simulink model "fcev_model_ssc"  (R2023a)
settings: Solver=VariableStepAuto  StartTime=0.0  StopTime=2474  RelTol=1e-3
model workspace (MAT data in the model file):
  N_P0 = 3
libraries: nesl_utility x12, fl_lib x7, sdl_lib x6, ee_lib x2, autolibshared x2, slpidlib x2, autolibdatasheetbattery x1, simulink x1, autolibmappedmotor x1
settings Model: Creator=connl  LastModifiedBy=connl
settings SolverCC: MaxConsecutiveMinStep=5  DaesscMode=Robust  SolverResetMethod=Robust
settings DebuggingCC: AlgebraicLoopMsg=none

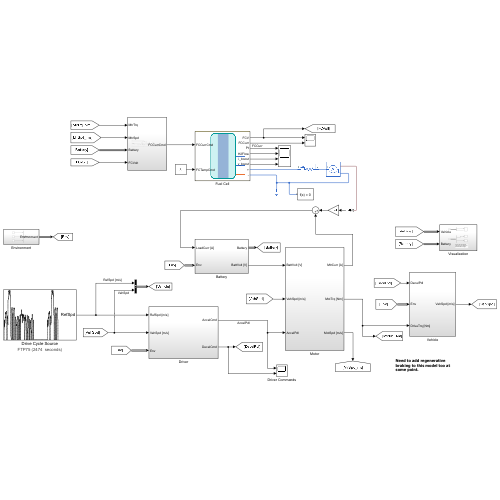
[thumbnail: Simulink's stored preview of the top-level diagram]
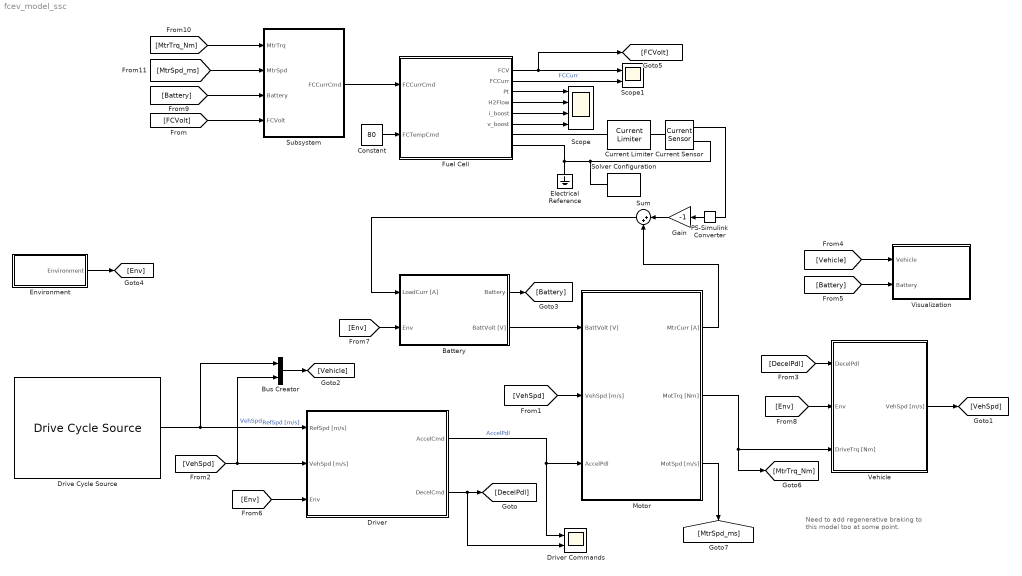
== system fcev_model_ssc ==
  note: Need to add regenerative braking to this model too at some point.
  Battery : Subsystem
  Bus Creator : BusCreator  Inputs=2
  Constant : Constant  Value=80
  Current Limiter : ee_lib/Semiconductors & Converters/Current Limiter  iLim=25 A  vLim=0.1 V  gLim=1e-3 1/Ohm  thermal_mass=100 J/K  initial_temperature=298.15 K
      settings: InternalSimscapePortConfiguration="{\"Bottom\":[],\"Left\":[{\"id\":\"p\",\"label\":\"+\",\"type\":\"foundation.electrical.electrical\"}],\"Right\":[{\"id\":\"n\",\"label\":\"-\",\"type\":\"foundation.electrical.electrical\"}],\"Top\":[]}"
  Current Sensor : fl_lib/Electrical/Electrical Sensors/Current Sensor
  Drive Cycle Source : autolibshared/Drive Cycle Source  cycleVar=FTP75  fileVar=cycleFTP75.mat  tfinal="2474  seconds"  cycleRepeat=off  outAccPort=off  outGearPort=off  gearList=No gear data  t_wot1=5  xdot_woto=0  xdot_wot1=30  t_wot2=20  xdot_wot2=0  t_wotend=30  srcUnit=m/s  outUnit=m/s  srcAccUnit=m/s/s  outAccUnit=m/s^2  dt=0  aMode=1  faultOption=off  velBnd=2  velBndUnit=mph  inUnit=m/s  timeBnd=1  failOption=off  stopSim=off  maxFaultCnt=10  maxFaultTime=2  maxTotFaultTime=15  traceOption=off  dtTrace=1  traceWindow=10  lastDCname=FTP75  lastOutUnit=mph  lastDT=0  lastTB=1  lastSB=2  forceCalcBound=off
  Driver : Subsystem
  Driver Commands : Scope  NumInputPorts=2
  Electrical Reference : fl_lib/Electrical/Electrical Elements/Electrical Reference
  Environment : Subsystem
  Fuel Cell : Subsystem  VariantControl=0
      mask Display: image('fuel_cell_converter_IMAGE.png'); % Use "Edit Image" on toolstrip to change.
  Gain : Gain  Gain=-1
  Motor : Subsystem
  PS-Simulink Converter : nesl_utility/PS-Simulink Converter  PhysicalDomain=network_engine_domain  SubClassName=ps_output  LeftPortType=input  RightPortType=output  PseudoPeriodic=off  Frequencies=[]  VectorFormat=inherit  Unit=inherit  AffineConversion=off
  Scope : Scope  NumInputPorts=4
  Scope1 : Scope  NumInputPorts=2
  Solver Configuration : nesl_utility/Solver Configuration  PhysicalDomain=network_engine_domain  SubClassName=solver  LeftPortType=input  RightPortType=generic  Tones=[]  Harmonics=[]  SimulateNoise=off  Profile=off  UseLocalSampling=off  EnableSwitchedLinearOptims=on  FrequencyDomain=off  UseCCode=off  RelTol=0.001  AbsTol=0.001  MinStep=1e-09  ToWorkspace=off  RevertToSquareIcSolve=off  NumHomotopyIterations=100  PhasorMode=off  PhasorModeNumHarmonics=1  ConsistencySolver=NEWTON_XTOL_AFTER_FTOL  IndexReductionMethod=DerivativeReplacement  DoDC=off  ResidualTolerance=1e-09  ConsistencyTolSource=GLOBAL  ConsistencyAbsTol=0.001  ConsistencyRelTol=0.001  ConsistencyTolFactor=0.001  UseLocalSolver=off  LocalSolverChoice=NE_BACKWARD_EULER_ADVANCER  ResolveIndetEquations=on  FunctionEvalNumThread=1  LocalSolverSampleTime=0.001  DoFixedCost=off  MaxNonlinIter=3  MaxModeIter=2  ComputeImpulses=off  ImpulseIterations=2  LinearAlgebra=auto  LinearAlgebraNumThread=0  EquationFormulation=NE_TIME_EF  DelaysMemoryBudget=1024  AutomaticFiltering=on  FilteringTimeConstant=0.001  PartitionStorageMethod=AS_NEEDED  PartitionMemoryBudget=1024  PartitionMethod=ROBUST
  Subsystem : Subsystem
  Sum : Sum  Inputs=|++
  Vehicle : Subsystem
  Visualization : Subsystem
  wires:
  Drive Cycle Source/1 -> Driver/1(RefSpd [m/s]), Bus Creator/1  "RefSpd [m/s]"
  Battery/2(BattVolt [V]) -> Motor/1(BattVolt [V])
  [VehSpd] -> Motor/2(VehSpd [m/s])
  [VehSpd] -> Driver/2(VehSpd [m/s]), Bus Creator/2  "VehSpd"
  [DecelPdl] -> Vehicle/1(DecelPdl)
  Vehicle/1(VehSpd [m/s]) -> [VehSpd]
  Bus Creator/1 -> [Vehicle]
  [Vehicle] -> Visualization/1(Vehicle)
  [Battery] -> Visualization/2(Battery)
  Environment/1(Environment) -> [Env]
  Battery/1(Battery) -> [Battery]
  Driver/1(AccelCmd) -> Driver Commands/1, Motor/3(AccelPdl)  "AccelPdl"
  Driver/2(DecelCmd) -> Driver Commands/2, [DecelPdl]
  [Env] -> Battery/2(Env)
  [Env] -> Driver/3(Env)
  [Env] -> Vehicle/2(Env)
  Motor/1(MtrCurr [A]) -> Sum/2
  Motor/2(MotTrq [Nm]) -> [MtrTrq_Nm], Vehicle/3(DriveTrq [Nm])
  Fuel Cell/4(H2Flow) -> Scope/2
  Fuel Cell/5(i_boost) -> Scope/3
  Fuel Cell/6(v_boost) -> Scope/4
  Fuel Cell/2(FCCurr) -> Scope1/2  "FCCurr"
  Sum/1 -> Battery/1(LoadCurr [A])
  Fuel Cell/3(Pt) -> Scope/1
  Fuel Cell/1(FCV) -> [FCVolt], Scope1/1
  Constant/1 -> Fuel Cell/2(FCTempCmd)
  Motor/3(MotSpd [m/s]) -> [MtrSpd_ms]
  [MtrTrq_Nm] -> Subsystem/1(MtrTrq)
  [MtrSpd_ms] -> Subsystem/2(MtrSpd)
  [Battery] -> Subsystem/3(Battery)
  [FCVolt] -> Subsystem/4(FCVolt)
  Subsystem/1(FCCurrCmd) -> Fuel Cell/1(FCCurrCmd)
  PS-Simulink Converter/1 -> Gain/1
  Gain/1 -> Sum/1
  connections:
  Fuel Cell/RConn1 -- Current Limiter/LConn1
  Fuel Cell/RConn2 -- Current Sensor/RConn2 -- Solver Configuration/RConn1 -- Electrical Reference/LConn1
  Current Sensor/RConn1 -- PS-Simulink Converter/LConn1
  Current Limiter/RConn1 -- Current Sensor/LConn1

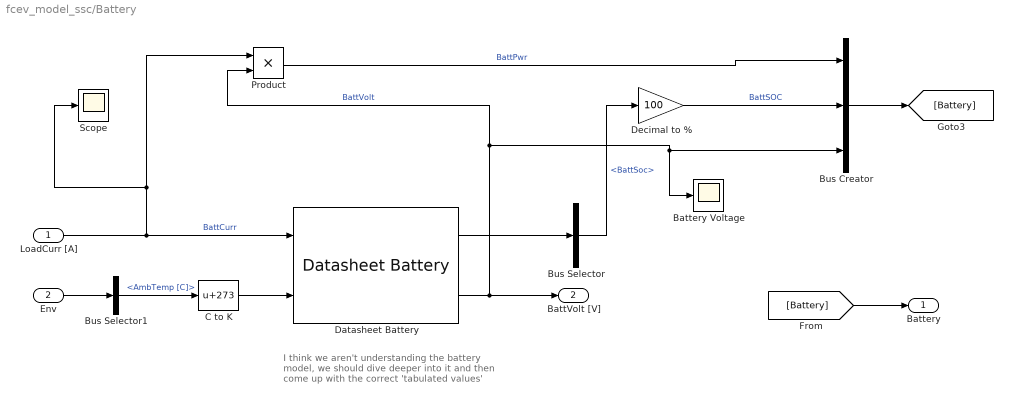
== system fcev_model_ssc/Battery ==
  note: I think we aren't understanding the battery model, we should dive deeper into it and then come up with the correct 'tabulated values'
  LoadCurr [A] : Inport
  Env : Inport  Port=2
  Battery Voltage : Scope
  Bus Creator : BusCreator  Inputs=3
  Bus Selector : BusSelector  OutputSignals=BattSoc
  Bus Selector1 : BusSelector  OutputSignals=AmbTemp [C]
  C to K : Bias  Bias=273  SaturateOnIntegerOverflow=off
  Datasheet Battery : autolibdatasheetbattery/Datasheet Battery  CapacityCtrl=Parameter  OutputVlt=Unfiltered  BattChargeMax=16  Em=[2.8 3.228 3.284 3.361 3.408 3.427 3.472 3.477 3.493 3.504 3.516 3.528 3.537 3.545 3.555 3.561 3.566 3.576 3.587 3.589 3.594 3.6 3.608 3.61 3.616 3.619 3.626 3.632 3.637 3.64 3.645 3.646 3.652 3.655 3.658 3.661 3.664 3.668 3.673 3.678 3.68 3.681 3.686 3.692 3.699 3.702 3.705 3.71 3.717 3.723 3.728 3.733 3.735 3.742 3.749 3.755 3.761 3.768 3.773 3.78 3.791 3.798 3.798 3.814 3.818 3.825 3.841 3.846 3.855 3.863 3.877 3.885 3.894 3.907 3.919 3.926 3.935 3.944 3.954 3.964 3.974 3.988 3.998 4.014 4.029 4.034 4.047 4.065 4.074 4.086 4.097 4.131 4.126 4.138 4.15 4.18 4.174 4.187 4.207 4.231 4.221]  CapLUTBp=[0 0.01 0.02 0.03 0.04 0.05 0.06 0.07 0.08 0.09 0.1 0.11 0.12 0.13 0.14 0.15 0.16 0.17 0.18 0.19 0.2 0.21 0.22 0.23 0.24 0.25 0.26 0.27 0.28 0.29 0.3 0.31 0.32 0.33 0.34 0.35 0.36 0.37 0.38 0.39 0.4 0.41 0.42 0.43 0.44 0.45 0.46 0.47 0.48 0.49 0.5 0.51 0.52 0.53 0.54 0.55 0.56 0.57 0.58 0.59 0.6 0.61 0.62 0.63 0.64 0.65 0.66 0.67 0.68 0.69 0.7 0.71 0.72 0.73 0.74 0.75 0.76 0.77 0.78 0.79 0.8 0.81 0.82 0.83 0.84 0.85 0.86 0.87 0.88 0.89 0.9 0.91 0.92 0.93 0.94 0.95 0.96 0.97 0.98 0.99 1]  RInt=0.001*[1, 1, 1, 1, 1, 1;1, 1, 1, 1, 1, 1]  BattTempBp=[240, 320]  CapSOCBp=[0 0.2 0.4 0.6 0.8 1]  Ns=12  Np=2  BattCapInit=32  Tc=1/1000  Vinit=4.221  RefBlkName='autolibdatasheetbattery/Datasheet Battery'
  Decimal to % : Gain  Gain=100
  Product : Product
  Scope : Scope
  Battery : Outport
  BattVolt [V] : Outport  Port=2
  wires:
  C to K/1 -> Datasheet Battery/2
  Datasheet Battery/1 -> Bus Selector/1
  Bus Selector/1 -> Decimal to %/1  "<BattSoc>"
  Decimal to %/1 -> Bus Creator/2  "BattSOC"
  Datasheet Battery/2 -> BattVolt [V]/1, Product/2, Bus Creator/3, Battery Voltage/1  "BattVolt"
  [Battery] -> Battery/1
  Env/1 -> Bus Selector1/1
  Bus Selector1/1 -> C to K/1  "<AmbTemp [C]>"
  Product/1 -> Bus Creator/1  "BattPwr"
  LoadCurr [A]/1 -> Scope/1, Product/1, Datasheet Battery/1  "BattCurr"
  Bus Creator/1 -> [Battery]

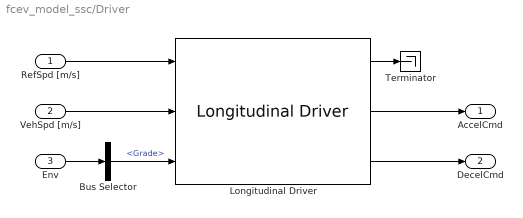
== system fcev_model_ssc/Driver ==
  RefSpd [m/s] : Inport
  VehSpd [m/s] : Inport  Port=2
  Env : Inport  Port=3
  Bus Selector : BusSelector  OutputSignals=Grade
  Longitudinal Driver : autolibshared/Longitudinal Driver  extAccelOvr=off  extDecelOvr=off  extAccelHld=off  extDecelHld=off  extAccelZero=off  extDecelZero=off  cntrlType=PI  shftType=None  velUnits=m/s  gearOut=off  Kp=20  Ki=1  Kff=.05  Kg=.01  VehVelVec=[0 100]  KffVec=[.1 .1]  KpVec=[10 10]  KiVec=[5 5]  KgVec=[0 0]  m=1500  Kpt=3000  tau=.1  L=2  aR=200  bR=2.5  cR=.5  g=9.81  vnom=100  Kaw=.1  tauerr=.03  tauPt=2  GearInit=0  tShift=.1  pdlVec=[0.1 0.4 0.5 0.9]  upShftTbl=[-1 12.9375 26.4375 39.9375 51.18749999999999 62.4375 72.84375 83.25;-1 16.3125 29.8125 43.3125 54.5624 65.8125 76.78125 87.75;-1 19.6875 33.1875 46.68749999999999 57.9375 69.1875 80.71875 92.25;-1 33 52.5 77.25 100.5 138.75 161.875 185]  dwnShftTbl=[1 9.5625 23.0625 36.5625 47.8125 59.0625 68.90625 78.75;1 12.9375 26.4375 39.9375 51.18749999999999 62.4375 72.84375 83.25;1 16.3125 29.8125 43.3125 54.562499 65.8125 76.78125 87.75;1 19.6875 33.1875 46.68749999999999 57.9375 69.1875 80.71875 92.25]  tClutch=.5  tRev=.5  tPark=120  aMode=1  UpGearVec="[0  1  2  3  4  5  6  7]"  DownGearVec="[1  2  3  4  5  6  7  8]"
  Terminator : Terminator
  AccelCmd : Outport
  DecelCmd : Outport  Port=2
  wires:
  VehSpd [m/s]/1 -> Longitudinal Driver/2
  Longitudinal Driver/2 -> AccelCmd/1
  RefSpd [m/s]/1 -> Longitudinal Driver/1
  Bus Selector/1 -> Longitudinal Driver/3  "<Grade>"
  Env/1 -> Bus Selector/1
  Longitudinal Driver/3 -> DecelCmd/1
  Longitudinal Driver/1 -> Terminator/1

== system fcev_model_ssc/Environment ==
  AmbTemp : Constant  Value=25
  Bus Creator : BusCreator  Inputs=3
  Grade : Constant  Value=0
  WindSpdx : Constant  Value=0
  Environment : Outport
  wires:
  Grade/1 -> Bus Creator/1  "Grade"
  WindSpdx/1 -> Bus Creator/2  "WindSpdx [m/s]"
  AmbTemp/1 -> Bus Creator/3  "AmbTemp [C]"
  Bus Creator/1 -> Environment/1

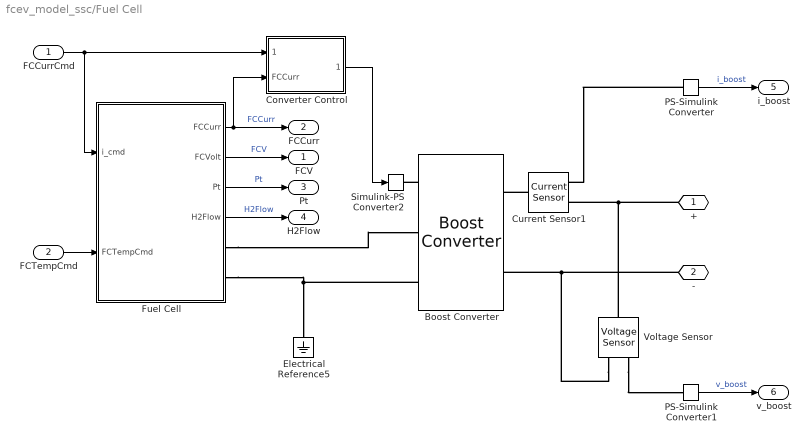
== system fcev_model_ssc/Fuel Cell ==
  FCCurrCmd : Inport
  FCTempCmd : Inport  Port=2
  Boost Converter : ee_lib/Semiconductors & Converters/Converters/Boost Converter  port_option=ee.enum.controlport.ps  device_type=ee.enum.converters.switchingdevice.averaged  Vf=0.8 V  Ron=0.001 Ohm  Rds=0.001 Ohm  Goff=1e-5 1/Ohm  Vgt=1 V  Vgt_off=-1 V  Ih=1 A  Vth=6 V  K=0  diode_param=ee.enum.converters.diode.nodynamics  diode_Vf=0.8 V  diode_Ron=0.001 Ohm  diode_Goff=1e-05 1/Ohm  diode_C=50 nF  diode_iRM=-235 A  diode_iF=300 A  diode_idot=-50 A/us  diode_trr_param=ee.enum.converters.diodetrr.trr_factor  diode_trr_factor=3  diode_trr=15 us  diode_Qrr=1500 s*uA  Lf=0.005 H  Rl=0 Ohm  Cf=0.001 F  Rf=10 Ohm  snubber_type=ee.enum.converters.snubber.exclude  Cs=1e-7 F  Rs=0.1 Ohm  iL_specify=on  iL_priority=High  iL=0 A  iL_nominal_specify=off  iL_nominal_unit=A  iL_nominal_value=1  vc_specify=on  vc_priority=High  vc=650 V  vc_nominal_specify=off  vc_nominal_unit=V  vc_nominal_value=1
      settings: InternalSimscapePortConfiguration="{\"Bottom\":[],\"Left\":[{\"id\":\"G\",\"label\":\"G\",\"type\":\"input\"},{\"id\":\"p1\",\"label\":\"1+\",\"type\":\"foundation.electrical.electrical\"},{\"id\":\"n1\",\"label\":\"1-\",\"type\":\"foundation.electrical.electrical\"}],\"Right\":[{\"id\":\"p2\",\"label\":\"2+\",\"type\":\"foundation.electrical.electrical\"},{\"id\":\"n2\",\"label\":\"2-\",\"type\":\"foundation.electrical.electrical\"}],\"Top\":[]}"
  Converter Control : Subsystem
  Current Sensor1 : fl_lib/Electrical/Electrical Sensors/Current Sensor
  Electrical Reference5 : fl_lib/Electrical/Electrical Elements/Electrical Reference
  Fuel Cell : Subsystem  Variant=on  VariantControlMode=label  VariantControl=Choice  LabelModeActiveChoice=SimscapeFuelCell
  PS-Simulink Converter : nesl_utility/PS-Simulink Converter  PhysicalDomain=network_engine_domain  SubClassName=ps_output  LeftPortType=input  RightPortType=output  PseudoPeriodic=off  Frequencies=[]  VectorFormat=inherit  Unit=inherit  AffineConversion=off
  PS-Simulink Converter1 : nesl_utility/PS-Simulink Converter  PhysicalDomain=network_engine_domain  SubClassName=ps_output  LeftPortType=input  RightPortType=output  PseudoPeriodic=off  Frequencies=[]  VectorFormat=inherit  Unit=inherit  AffineConversion=off
  Simulink-PS Converter2 : nesl_utility/Simulink-PS Converter  PhysicalDomain=network_engine_domain  SubClassName=ps_input  LeftPortType=input  RightPortType=output  PseudoPeriodic=off  Frequencies=[]  NoiseDistribution=none  NoiseParameters=[]  Unit=1  AffineConversion=off  FilteringAndDerivatives=provide  SimscapeFilterOrder=1  InputFilterTimeConstant=0.001  UdotUserProvided=0
  Voltage Sensor : fl_lib/Electrical/Electrical Sensors/Voltage Sensor
  + : PMIOPort  Side=Right
  - : PMIOPort  Port=2  Side=Right
  FCV : Outport
  FCCurr : Outport  Port=2
  Pt : Outport  Port=3
  H2Flow : Outport  Port=4
  i_boost : Outport  Port=5
  v_boost : Outport  Port=6
  wires:
  Converter Control/1(u_boost) -> Simulink-PS Converter2/1
  Fuel Cell/1(FCCurr) -> FCCurr/1, Converter Control/2(FCCurr)  "FCCurr"
  FCCurrCmd/1 -> Fuel Cell/1(i_cmd), Converter Control/1(FCCurrCmd)
  FCTempCmd/1 -> Fuel Cell/2(FCTempCmd)
  Fuel Cell/2(FCVolt) -> FCV/1  "FCV"
  Fuel Cell/3(Pt) -> Pt/1  "Pt"
  Fuel Cell/4(H2Flow) -> H2Flow/1  "H2Flow"
  PS-Simulink Converter/1 -> i_boost/1  "i_boost"
  PS-Simulink Converter1/1 -> v_boost/1  "v_boost"
  connections:
  Boost Converter/LConn1 -- Simulink-PS Converter2/RConn1
  -/RConn1 -- Voltage Sensor/RConn2 -- Boost Converter/RConn2
  +/RConn1 -- Voltage Sensor/LConn1 -- Current Sensor1/RConn2
  Current Sensor1/LConn1 -- Boost Converter/RConn1
  Boost Converter/LConn3 -- Fuel Cell/RConn2 -- Electrical Reference5/LConn1
  PS-Simulink Converter/LConn1 -- Current Sensor1/RConn1
  Fuel Cell/RConn1 -- Boost Converter/LConn2
  Voltage Sensor/RConn1 -- PS-Simulink Converter1/LConn1

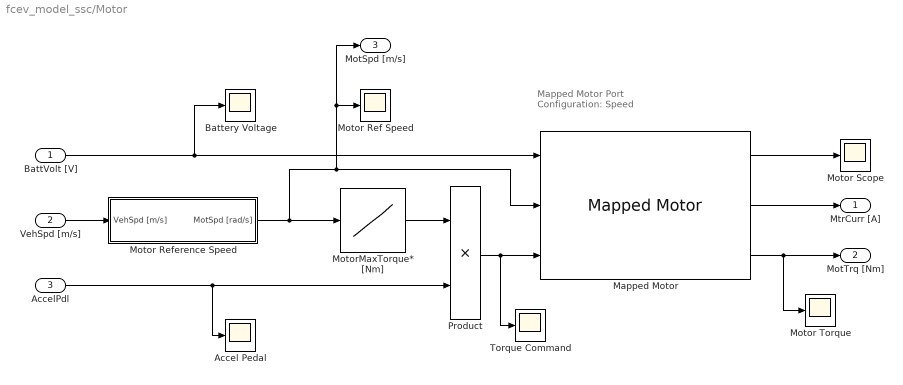
== system fcev_model_ssc/Motor ==
  note: Mapped Motor
      | Port Configuration: Speed
  BattVolt [V] : Inport
  VehSpd [m/s] : Inport  Port=2
  AccelPdl : Inport  Port=3
  Accel Pedal : Scope
  Battery Voltage : Scope
  Mapped Motor : autolibmappedmotor/Mapped Motor  port_config=Speed  param_by=Tabulated torque-speed envelope  w_t=[0, 100, 200, 300, 400, 500, 600]  T_t=[85, 85, 85, 80, 70, 55, 30]  torque_max=110  power_max=21000  Tc=0.02  param_loss=Single efficiency measurement  eff=90  w_eff=400  T_eff=55  Piron=0  Pbase=0  w_eff_bp=[-800 -400 0 400 800]  T_eff_bp=[0 0.03 0.06 0.09]  Temp_eff_bp=[233.15 293.15 373.15]  losses_table=[1.49 1.67 2.21 3.10; 0.42 0.69 1.14 2.03; 0.06 0.24 0.78 1.68; 0.42 0.69 1.14 2.03; 1.49 1.67 2.21 3.10]  losses_table_3d=cat(3,[1.49 1.67 2.21 3.10; 0.42 0.69 1.14 2.03; 0.06 0.24 0.78 1.68; 0.42 0.69 1.14 2.03; 1.49 1.67 2.21 3.10],[1.49 1.67 2.21 3.10; 0.42 0.69 1.14 2.03; 0.06 0.24 0.78 1.68; 0.42 0.69 1.14 2.03; 1.49 1.67 2.21 3.10],[1.49 1.67 2.21 3.10; 0.42 0.69 1.14 2.03; 0.06 0.24 0.78 1.68; 0.42 0.69 1.14 2.03; 1.49 1.67 2.21 3.10])  efficiency_table=[95 95 95 95; 95 95 95 95; 95 95 95 95; 95 95 95 95; 95 95 95 95]  efficiency_table_3d=cat(3,[95 95 95 95; 95 95 95 95; 95 95 95 95; 95 95 95 95; 95 95 95 95],[95 95 95 95; 95 95 95 95; 95 95 95 95; 95 95 95 95; 95 95 95 95],[95 95 95 95; 95 95 95 95; 95 95 95 95; 95 95 95 95; 95 95 95 95])  J=5e-6  b=1e-5  omega_o=0  T_t_extended=[30 55 70 80 85 85 85 85 85 80 70 55 30]  w_t_extended=[-600 -500 -400 -300 -200 -100 0 100 200 300 400 500 600]  KLossIron=0  KLossCopper=0.80808  x_w_eff_vec=[-8000 -4000 0 4000 8000]  x_T_eff_vec=[-0.09 -0.06 -0.03 0 0.03 0.06 0.09]  x_tmp_eff_vec=[-0.09 -0.06 -0.03 0 0.03 0.06 0.09]  x_losses_mat=[3.1 2.21 1.67 1.49 1.67 2.21 3.1;2.03 1.14 0.69 0.42 0.69 1.14 2.03;1.68 0.78 0.24 0.06 0.24 0.78 1.68;2.03 1.14 0.69 0.42 0.69 1.14 2.03;3.1 2.21 1.67 1.49 1.67 2.21 3.1]  x_losses_mat_3d=[37.8947368421052 25.2631578947368 12.6315789473684 0 12 24 36;18.9473684210526 12.6315789473684 6.3157894736842 0 5.99999999999999 12 18;0 0 0 0 0 0 0;18 12 5.99999999999999 0 6.3157894736842 12.6315789473684 18.9473684210526;36 24 12 0 12.6315789473684 25.2631578947368 37.8947368421052]  CalLossMapData={}  CalLossWithTempMapData={}  aMode=1  RefBlkName='autolibmappedmotor/Mapped Motor'
      settings: LibrarySourceBlock=autolibemachines/Mapped Motor
  Motor Ref Speed : Scope
  Motor Reference Speed : Subsystem
  Motor Scope : Scope
  Motor Torque : Scope
  MotorMaxTorque* [Nm] : Lookup_n-D  NumberOfTableDimensions=1  BreakpointsForDimension1=[0, 100, 200, 300, 400, 500, 600]  Table=[85, 85, 85, 80, 70, 55, 30]  InternalRulePriority=Speed  RndMeth=Simplest
  Product : Product
  Torque Command : Scope
  MtrCurr [A] : Outport
  MotTrq [Nm] : Outport  Port=2
  MotSpd [m/s] : Outport  Port=3
  wires:
  VehSpd [m/s]/1 -> Motor Reference Speed/1(VehSpd [m/s])
  MotorMaxTorque* [Nm]/1 -> Product/1
  AccelPdl/1 -> Accel Pedal/1, Product/2
  Product/1 -> Torque Command/1, Mapped Motor/3
  BattVolt [V]/1 -> Battery Voltage/1, Mapped Motor/1
  Mapped Motor/2 -> MtrCurr [A]/1
  Mapped Motor/3 -> Motor Torque/1, MotTrq [Nm]/1
  Motor Reference Speed/1(MotSpd [rad/s]) -> Mapped Motor/2, MotSpd [m/s]/1, Motor Ref Speed/1, MotorMaxTorque* [Nm]/1
  Mapped Motor/1 -> Motor Scope/1

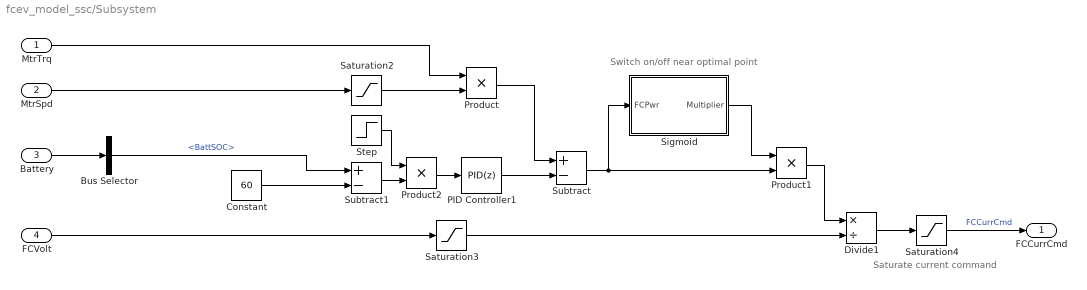
== system fcev_model_ssc/Subsystem ==
  note: Switch on/off near optimal point
  note: Saturate current command
  MtrTrq : Inport
  MtrSpd : Inport  Port=2
  Battery : Inport  Port=3
  FCVolt : Inport  Port=4
  Bus Selector : BusSelector  OutputSignals=BattSOC
  Constant : Constant  Value=60
  Divide1 : Product  Inputs=*/
  PID Controller1 : slpidlib/PID Controller  Controller=PID  Form=Parallel  TimeDomain=Discrete-time  UseExternalTs=off  SampleTime=-1  IntegratorMethod=Forward Euler  FilterMethod=Forward Euler  ControllerParametersSource=internal  P=10000/2  I=0  UseKiTs=off  D=0  N=100  UseFilter=on  TunerSelectOption=Transfer Function Based (PID Tuner App)  ZeroCross=off  InitialConditionSource=internal  InitialConditionForIntegrator=0  InitialConditionForFilter=0  DifferentiatorICPrevScaledInput=0  ExternalReset=none  TrackingMode=off  Kt=1  LimitOutput=off  SatLimitsSource=internal  UpperSaturationLimit=inf  LowerSaturationLimit=-inf  LinearizeAsGain=on  AntiWindupMode=none  Kb=1  LimitIntegrator=off  UpperIntegratorSaturationLimit=inf  LowerIntegratorSaturationLimit=-inf  POutMin=[]  POutMax=[]  IOutMin=[]  IOutMax=[]  DOutMin=[]  DOutMax=[]  NOutMin=[]  NOutMax=[]  SumOutMin=[]  SumOutMax=[]  SaturationOutMin=[]  SaturationOutMax=[]  PParamMin=[]  PParamMax=[]  IParamMin=[]  IParamMax=[]  DParamMin=[]  DParamMax=[]  NParamMin=[]  NParamMax=[]  KbParamMin=[]  KbParamMax=[]  KtParamMin=[]  KtParamMax=[]  KbOutMin=[]  KbOutMax=[]  KtOutMin=[]  KtOutMax=[]  IntegratorOutMin=[]  IntegratorOutMax=[]  FilterOutMin=[]  FilterOutMax=[]  SumI1OutMin=[]  SumI1OutMax=[]  SumI2OutMin=[]  SumI2OutMax=[]  SumI3OutMin=[]  SumI3OutMax=[]  SumI4OutMin=[]  SumI4OutMax=[]  SumDOutMin=[]  SumDOutMax=[]  DifferentiatorOutMin=[]  DifferentiatorOutMax=[]  FilterDiffOutCoefMin=[]  FilterDiffOutCoefMax=[]  ReciprocalOutMin=[]  ReciprocalOutMax=[]  SumDenOutMin=[]  SumDenOutMax=[]  SumNumOutMin=[]  SumNumOutMax=[]  DivideOutMin=[]  DivideOutMax=[]  UdiffTsProdOutMin=[]  UdiffTsProdOutMax=[]  NTsProdOutMin=[]  NTsProdOutMax=[]  UintegralTsProdOutMin=[]  UintegralTsProdOutMax=[]  UngainTsProdOutMin=[]  UngainTsProdOutMax=[]  ClampingZeroOutDataTypeStr=Inherit: Inherit via back propagation  ClampingZeroOutMin=[]  ClampingZeroOutMax=[]  FilterDenConstantOutDataTypeStr=Inherit: Inherit via back propagation  FilterDenConstantOutMin=[]  FilterDenConstantOutMax=[]  PCopyOutDataTypeStr=Inherit: Inherit via back propagation  PCopyOutMin=[]  PCopyOutMax=[]  NCopyOutDataTypeStr=Inherit: Inherit via back propagation  NCopyOutMin=[]  NCopyOutMax=[]  IntegratorContinuousStateAttributes=''  IntegratorStateMustResolveToSignalObject=off  IntegratorRTWStateStorageClass=Auto  FilterContinuousStateAttributes=''  FilterStateMustResolveToSignalObject=off  FilterRTWStateStorageClass=Auto  ParallelPVariant=InternalParameters  IdealPVariant=Disabled  IVariant=InternalParameters  DVariant=InternalParameters  IntegratorVariant=Discrete  SatVariant=Disabled  AWVariant=Passthrough  PCopyVariant=Disabled  TRVariant=Disabled  FdbkBlocksVariant=Forward  IdealPFdbkVariant=Disabled  SatFdbkVariant=Disabled  DerivativeFilterVariant=ForwardEulerFilter  NVariant=InternalParameters  NCopyVariant=Disabled  FilterICVariant=InternalICsFilter  IntegratorICVariant=InternalICs  ExternalResetVariant=Disabled  TRSumVariant=Passthrough  SumFdbkVariant=Disabled  SumVariant=Sum_PID  TsampFilterVariant=InternalTs  TsampNgainVariant=Passthrough  TsampIntegralVariant=Disabled_SignalSpec  ExternalSaturationOutDataTypeStr=Inherit: Same as second input
  Product : Product
  Product1 : Product
  Product2 : Product
  Saturation2 : Saturate  UpperLimit=inf  LowerLimit=1  ZeroCross=off
  Saturation3 : Saturate  UpperLimit=inf  LowerLimit=200  ZeroCross=off
  Saturation4 : Saturate  UpperLimit=350  LowerLimit=0  ZeroCross=off
  Sigmoid : Subsystem
  Step : Step  SampleTime=0.01
  Subtract : Sum  Inputs=+-
  Subtract1 : Sum  Inputs=+-
  FCCurrCmd : Outport  SampleTime=.01
  wires:
  Step/1 -> Product2/1
  Constant/1 -> Subtract1/2
  Product1/1 -> Divide1/1
  Saturation3/1 -> Divide1/2
  Saturation4/1 -> FCCurrCmd/1  "FCCurrCmd"
  Subtract/1 -> Product1/2, Sigmoid/1(FCPwr)
  Product/1 -> Subtract/1
  Divide1/1 -> Saturation4/1
  Saturation2/1 -> Product/2
  PID Controller1/1 -> Subtract/2
  Sigmoid/1(Multiplier) -> Product1/1
  Subtract1/1 -> Product2/2
  MtrTrq/1 -> Product/1
  Product2/1 -> PID Controller1/1
  MtrSpd/1 -> Saturation2/1
  FCVolt/1 -> Saturation3/1
  Battery/1 -> Bus Selector/1
  Bus Selector/1 -> Subtract1/1  "<BattSOC>"

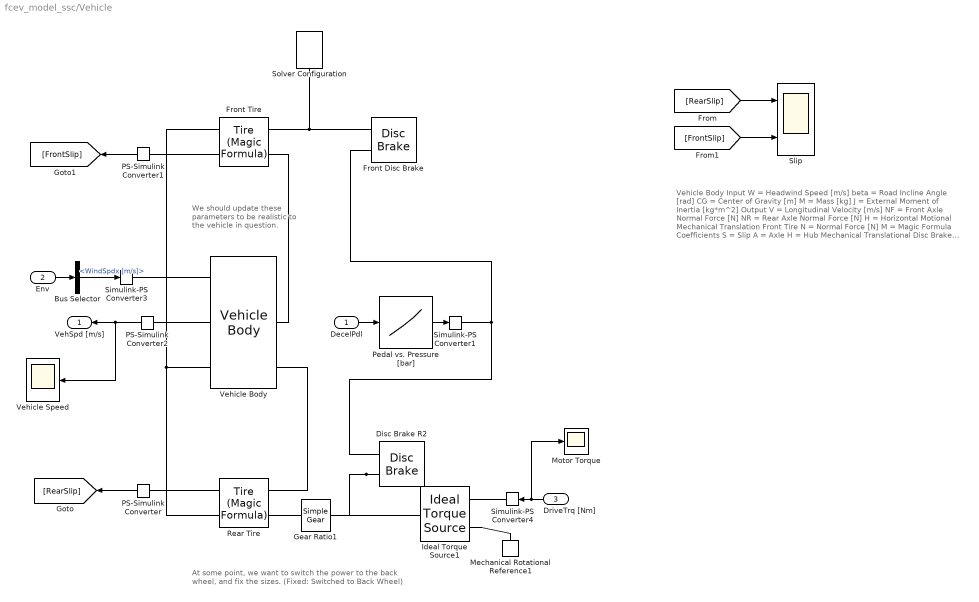
== system fcev_model_ssc/Vehicle ==
  note: We should update these parameters to be realistic to the vehicle in question.
  note: Vehicle Body
      | Input
      | W = Headwind Speed [m/s]
      | beta = Road Incline Angle [rad]
      | CG = Center of Gravity [m]
      | M = Mass [kg]
      | J = External Moment of Inertia [kg*m^2]
      |
      | Output
      | V = Longitudinal Velocity [m/s]
      | NF = Front Axle Normal Force [N]
      | NR = Rear Axle Normal Force [N]
      | H = Horizontal Motional Mechanical Translation
      |
      | Front Tire
      | N = Normal Force [N]
      | M = Magic Formula Coefficients
      | S = Slip
      | A = Axle
      | H = Hub Mechanical Translational
      |
      | Disc Brake
      | P = Cylinder Pressure [bars]
      | S = Shaft Rotational Mechanical
      |
      | Ideal Torque Source
      | S = Control Signal [Nm]
      | C = Case Mechanical Rotational with the Source Reference Point
      | R = Rod Mechanical Rotational Port with the Source Moving Part
  note: At some point, we want to switch the power to the back wheel, and fix the sizes.
      | (Fixed: Switched to Back Wheel)
  DecelPdl : Inport
  Env : Inport  Port=2
  DriveTrq [Nm] : Inport  Port=3
  Bus Selector : BusSelector  OutputSignals=WindSpdx [m/s]
  Disc Brake R2 : sdl_lib/Brakes & Detents/Rotational/Disc Brake  r_mean=0.05 m  bore=0.05 m  n_pads=2  thermal_port=simscape.enum.thermaleffects.omit  mu_static=0.1  mu_coulomb=0.1  temperature_TLU=[280, 300, 320] K  mu_static_TLU=[.9, .8, .7]  mu_coulomb_TLU=[.8, .7, .6]  brkwy_vel=0.1 rad/s  visc_coef=0.001 N*m/(rad/s)  enable_faults=simscape.enum.onoff.off  faulted_pressure=0 bar  external_fault=simscape.enum.onoff.off  temporal_fault=simscape.enum.onoff.off  fault_time=5 s  report_fault=simscape.enum.assert.action.none  thermal_mass=50 kJ/K  temperature_specify=off  temperature_priority=High  temperature=300 K  temperature_nominal_specify=off  temperature_nominal_unit=K  temperature_nominal_value=1
  Front Disc Brake : sdl_lib/Brakes & Detents/Rotational/Disc Brake  r_mean=0.125 m  bore=0.125 m  n_pads=2  thermal_port=simscape.enum.thermaleffects.omit  mu_static=0.1  mu_coulomb=0.1  temperature_TLU=[280, 300, 320] K  mu_static_TLU=[.9, .8, .7]  mu_coulomb_TLU=[.8, .7, .6]  brkwy_vel=0.1 rad/s  visc_coef=0.001 N*m/(rad/s)  enable_faults=simscape.enum.onoff.off  faulted_pressure=0 bar  external_fault=simscape.enum.onoff.off  temporal_fault=simscape.enum.onoff.off  fault_time=5 s  report_fault=simscape.enum.assert.action.none  thermal_mass=50 kJ/K  temperature_specify=off  temperature_priority=High  temperature=300 K  temperature_nominal_specify=off  temperature_nominal_unit=K  temperature_nominal_value=1
  Front Tire : sdl_lib/Tires & Vehicles/Tire (Magic Formula)  parameterization=sdl.enum.magic_tire_model.peak  F_z1=3000 N  F_x1=3500 N  kappa1=6  B_m=10  C_m=1.9  D_m=1  E_m=0.97  fz0=4e+3 N  p_Cx=1.685  p_Dx=[ 1.21 -0.037 ]  p_Ex=[ 0.344 0.095 -0.02 0 ]  p_Kx=[ 21.51 -0.163 0.245 ]  p_Hx=[ -0.002 0.002 ]  p_Vx=[ 0 0 ]  rolling_radius_model=sdl.enum.RollingRadiusParameterization.Constant  r_e=0.31 m  r_0=0.3 m  breff=8.39  dreff=0.26  freff=0.074  q_re0=0.99  q_v1=0.008  longvl=17 m/s  cz=5e5 N/m  model_resistance=1  resistance_model=1  coeff=0.015  p_tire=250e3 Pa  alpha=-0.003  beta=0.97  coeff_a=84e-4  coeff_b=6.2e-4 s/m  coeff_c=1.6e-4 s^2/m^2  p_tire0=240e3 Pa  fz0_resistance=4000 N  vH0=16 m/s  q_Sy=[.0082, 0, .0014, .001, 0, 0, 1.08, -.5]  v_thr=1e-3 m/s  enable_scaling_coefficients=false  lfzO=1  lcx=1  lmux=1  lex=1  lkx=1  lhx=1  lvx=1  lmy=1  model_compliance=0  stiffness=1e+6 N/m  damping=1000 N/(m/s)  model_inertia=1  inertia=5 kg*m^2  initial_velocity=0 rad/s  vxlow=0.1 m/s  v_tr_thr=0.1*(0.1) m/s  kpumin=-1e5  kpumax=1e5
  Gear Ratio1 : sdl_lib/Gears/Simple Gear  ratio=1/3.2  rotation_direction=sdl.enum.shaftOutputDirection.same  friction_model=sdl.enum.gear_efficiencies_load.off  T_noload=0.1 N*m  T_nom=5 N*m  efficiency_nom=0.8  efficiency=0.8  temperature_TLU=[280, 300, 320] K  load_TLU=[1, 5, 10] N*m  efficiency_TLU=[.95, .9, .85]  efficiency_TLU2=[.85, .8, .75; .95, .9, .85; .85, .8, .7]  w_thr=0.01 rad/s  pwr_thr=0.001 W  enable_backlash=false  hardstop_model=simscape.enum.hardstop.smooth  backlash_distance=1e-3 mm  r_base=0.1 m  transition=1e-4 mm  backlash_stiffness=1e6 N/m  backlash_damping=1e3 N*s/m  coeff_rest=0.7  v_tol=0.001 m/s  f_tol=0.001 N  mu_visc=[0, 0] N*m*s/rad  enable_faults=simscape.enum.onoff.off  efficiency_fault=0.05  external_fault=simscape.enum.onoff.off  temporal_fault=simscape.enum.onoff.off  fault_time=5 s  fault_angles=pi / 12 rad  report_fault=simscape.enum.assert.action.none  thermal_mass=50 J/K  temperature_specify=off  temperature_priority=High  temperature=300 K  temperature_nominal_specify=off  temperature_nominal_unit=K  temperature_nominal_value=1  x_backlash_specify=off  x_backlash_priority=None  x_backlash=0 mm  x_backlash_nominal_specify=off  x_backlash_nominal_unit=mm  x_backlash_nominal_value=1  f_hardstop_specify=off  f_hardstop_priority=None  f_hardstop=0 N  f_hardstop_nominal_specify=off  f_hardstop_nominal_unit=N  f_hardstop_nominal_value=1  v_backlash_specify=off  v_backlash_priority=None  v_backlash=0 m/s  v_backlash_nominal_specify=off  v_backlash_nominal_unit=m/s  v_backlash_nominal_value=1
  Ideal Torque Source1 : fl_lib/Mechanical/Mechanical Sources/Ideal Torque Source
  Mechanical Rotational Reference1 : fl_lib/Mechanical/Rotational Elements/Mechanical Rotational Reference
  Motor Torque : Scope
  PS-Simulink Converter : nesl_utility/PS-Simulink Converter  PhysicalDomain=network_engine_domain  SubClassName=ps_output  LeftPortType=input  RightPortType=output  PseudoPeriodic=off  Frequencies=[]  VectorFormat=inherit  Unit=inherit  AffineConversion=off
  PS-Simulink Converter1 : nesl_utility/PS-Simulink Converter  PhysicalDomain=network_engine_domain  SubClassName=ps_output  LeftPortType=input  RightPortType=output  PseudoPeriodic=off  Frequencies=[]  VectorFormat=inherit  Unit=inherit  AffineConversion=off
  PS-Simulink Converter2 : nesl_utility/PS-Simulink Converter  PhysicalDomain=network_engine_domain  SubClassName=ps_output  LeftPortType=input  RightPortType=output  PseudoPeriodic=off  Frequencies=[]  VectorFormat=inherit  Unit=m/s  AffineConversion=off
  Pedal vs. Pressure [bar] : Lookup_n-D  NumberOfTableDimensions=1  BreakpointsForDimension1=[-5:5]  Table=tanh([-5:5])  InternalRulePriority=Speed  RndMeth=Simplest
  Rear Tire : sdl_lib/Tires & Vehicles/Tire (Magic Formula)  parameterization=1  F_z1=3000 N  F_x1=3500 N  kappa1=6  B_m=10  C_m=1.9  D_m=1  E_m=0.97  fz0=4e+3 N  p_Cx=1.685  p_Dx=[ 1.21 -0.037 ]  p_Ex=[ 0.344 0.095 -0.02 0 ]  p_Kx=[ 21.51 -0.163 0.245 ]  p_Hx=[ -0.002 0.002 ]  p_Vx=[ 0 0 ]  rolling_radius_model=sdl.enum.RollingRadiusParameterization.Constant  r_e=0.31 m  r_0=0.3 m  breff=8.39  dreff=0.26  freff=0.074  q_re0=0.99  q_v1=0.008  longvl=17 m/s  cz=5e5 N/m  model_resistance=1  resistance_model=1  coeff=0.015  p_tire=250e3 Pa  alpha=-0.003  beta=0.97  coeff_a=84e-4  coeff_b=6.2e-4 s/m  coeff_c=1.6e-4 s^2/m^2  p_tire0=240e3 Pa  fz0_resistance=4000 N  vH0=16 m/s  q_Sy=[.0082, 0, .0014, .001, 0, 0, 1.08, -.5]  v_thr=1e-3 m/s  enable_scaling_coefficients=false  lfzO=1  lcx=1  lmux=1  lex=1  lkx=1  lhx=1  lvx=1  lmy=1  model_compliance=0  stiffness=1e+6 N/m  damping=1000 N/(m/s)  model_inertia=1  inertia=5 kg*m^2  initial_velocity=0 rad/s  vxlow=0.1 m/s  v_tr_thr=0.1*(0.1) m/s  kpumin=-1e5  kpumax=1e5
  Simulink-PS Converter1 : nesl_utility/Simulink-PS Converter  PhysicalDomain=network_engine_domain  SubClassName=ps_input  LeftPortType=input  RightPortType=output  PseudoPeriodic=off  Frequencies=[]  NoiseDistribution=none  NoiseParameters=[]  Unit=bar  AffineConversion=off  FilteringAndDerivatives=provide  SimscapeFilterOrder=1  InputFilterTimeConstant=0.01  UdotUserProvided=0
  Simulink-PS Converter3 : nesl_utility/Simulink-PS Converter  PhysicalDomain=network_engine_domain  SubClassName=ps_input  LeftPortType=input  RightPortType=output  PseudoPeriodic=off  Frequencies=[]  NoiseDistribution=none  NoiseParameters=[]  Unit=m/s  AffineConversion=off  FilteringAndDerivatives=provide  SimscapeFilterOrder=1  InputFilterTimeConstant=0.01  UdotUserProvided=0
  Simulink-PS Converter4 : nesl_utility/Simulink-PS Converter  PhysicalDomain=network_engine_domain  SubClassName=ps_input  LeftPortType=input  RightPortType=output  PseudoPeriodic=off  Frequencies=[]  NoiseDistribution=none  NoiseParameters=[]  Unit=N*m  AffineConversion=off  FilteringAndDerivatives=provide  SimscapeFilterOrder=1  InputFilterTimeConstant=0.01  UdotUserProvided=0
  Slip : Scope  NumInputPorts=2
  Solver Configuration : nesl_utility/Solver Configuration  PhysicalDomain=network_engine_domain  SubClassName=solver  LeftPortType=input  RightPortType=generic  Tones=[]  Harmonics=[]  SimulateNoise=off  Profile=off  UseLocalSampling=off  EnableSwitchedLinearOptims=on  FrequencyDomain=off  UseCCode=off  RelTol=0.001  AbsTol=0.001  MinStep=1e-09  ToWorkspace=off  RevertToSquareIcSolve=off  NumHomotopyIterations=100  PhasorMode=off  PhasorModeNumHarmonics=1  ConsistencySolver=NEWTON_XTOL_AFTER_FTOL  IndexReductionMethod=DerivativeReplacement  DoDC=off  ResidualTolerance=1e-09  ConsistencyTolSource=GLOBAL  ConsistencyAbsTol=0.001  ConsistencyRelTol=0.001  ConsistencyTolFactor=0.001  UseLocalSolver=off  LocalSolverChoice=NE_BACKWARD_EULER_ADVANCER  ResolveIndetEquations=on  FunctionEvalNumThread=1  LocalSolverSampleTime=0.001  DoFixedCost=off  MaxNonlinIter=3  MaxModeIter=2  ComputeImpulses=off  ImpulseIterations=2  LinearAlgebra=auto  LinearAlgebraNumThread=0  EquationFormulation=NE_TIME_EF  DelaysMemoryBudget=1024  AutomaticFiltering=on  FilteringTimeConstant=0.001  PartitionStorageMethod=AS_NEEDED  PartitionMemoryBudget=1024  PartitionMethod=ROBUST
  Vehicle Body : sdl_lib/Tires & Vehicles/Vehicle Body  mass=200 kg  n_w=1  x_f=0.5 m  x_r=0.5 m  y_c=0.5 m  mass_var=simscape.enum.onoff.off  g=9.81 m/s^2  liftoff_warning=0  area=1 m^2  Cd=1.2  rho=1.18 kg/m^3  model_pitch=simscape.enum.onoff.off  inertia=4000 kg*m^2  suspension_model=1  k_f=1e4 N/m  b_f=1e4 N/(m/s)  k_r=1e4 N/m  b_r=1e4 N/(m/s)  k_f_TLU=[-2000, -1000, 0, 1000, 2000] N  x_f_TLU=[-.4, -.2, 0, .2, .4] m  b_f_TLU=[-200, -100, 0, 100, 200] N  v_f_TLU=[-4, -2, 0, 2, 4] m/s  k_r_TLU=[-2000, -1000, 0, 1000, 2000] N  x_r_TLU=[-.4, -.2, 0, .2, .4] m  b_r_TLU=[-200, -100, 0, 100, 200] N  v_r_TLU=[-4, -2, 0, 2, 4] m/s  interp_method=simscape.enum.interpolation.linear  extrap_method=simscape.enum.extrapolation.linear  model_hardstop=0  upper_bound_f=.25 m  lower_bound_f=-.25 m  stop_k_f=1e6 N/m  stop_b_f=150 N/(m/s)  upper_bound_r=.25 m  lower_bound_r=-.25 m  stop_k_r=1e6 N/m  stop_b_r=150 N/(m/s)  initial_pitch=0 rad  initial_pitch_rate=0 rad/s  v_specify=on  v_priority=High  v=0 m/s  v_nominal_specify=off  v_nominal_unit=m/s  v_nominal_value=1
  Vehicle Speed : Scope
  VehSpd [m/s] : Outport
  wires:
  PS-Simulink Converter/1 -> [RearSlip]
  [RearSlip] -> Slip/1
  PS-Simulink Converter1/1 -> [FrontSlip]
  [FrontSlip] -> Slip/2
  DecelPdl/1 -> Pedal vs. Pressure [bar]/1
  PS-Simulink Converter2/1 -> Vehicle Speed/1, VehSpd [m/s]/1
  Bus Selector/1 -> Simulink-PS Converter3/1  "<WindSpdx [m/s]>"
  Pedal vs. Pressure [bar]/1 -> Simulink-PS Converter1/1
  Env/1 -> Bus Selector/1
  DriveTrq [Nm]/1 -> Motor Torque/1, Simulink-PS Converter4/1
  connections:
  Rear Tire/RConn1 -- PS-Simulink Converter/LConn1
  Front Tire/RConn1 -- PS-Simulink Converter1/LConn1
  Vehicle Body/LConn1 -- Rear Tire/RConn2 -- Front Tire/RConn2
  Vehicle Body/RConn1 -- Rear Tire/LConn1
  Vehicle Body/RConn2 -- Front Tire/LConn1
  Disc Brake R2/LConn2 -- Gear Ratio1/RConn1 -- Ideal Torque Source1/LConn1
  Simulink-PS Converter1/RConn1 -- Front Disc Brake/LConn1 -- Disc Brake R2/LConn1
  Vehicle Body/LConn2 -- PS-Simulink Converter2/LConn1
  Simulink-PS Converter3/RConn1 -- Vehicle Body/LConn3
  Front Disc Brake/LConn2 -- Solver Configuration/RConn1 -- Front Tire/LConn2
  Ideal Torque Source1/RConn2 -- Mechanical Rotational Reference1/LConn1
  Ideal Torque Source1/RConn1 -- Simulink-PS Converter4/RConn1
  Rear Tire/LConn2 -- Gear Ratio1/LConn1

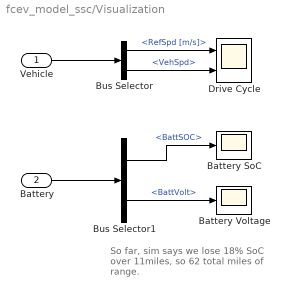
== system fcev_model_ssc/Visualization ==
  note: So far, sim says we lose 18% SoC over 11miles, so 62 total miles of range.
  Vehicle : Inport
  Battery : Inport  Port=2
  Battery SoC : Scope
  Battery Voltage : Scope
  Bus Selector : BusSelector  OutputSignals=RefSpd [m/s],VehSpd
  Bus Selector1 : BusSelector  OutputSignals=BattSOC,BattVolt
  Drive Cycle : Scope  NumInputPorts=2
  wires:
  Vehicle/1 -> Bus Selector/1
  Battery/1 -> Bus Selector1/1
  Bus Selector/1 -> Drive Cycle/1  "<RefSpd [m/s]>"
  Bus Selector/2 -> Drive Cycle/2  "<VehSpd>"
  Bus Selector1/1 -> Battery SoC/1  "<BattSOC>"
  Bus Selector1/2 -> Battery Voltage/1  "<BattVolt>"

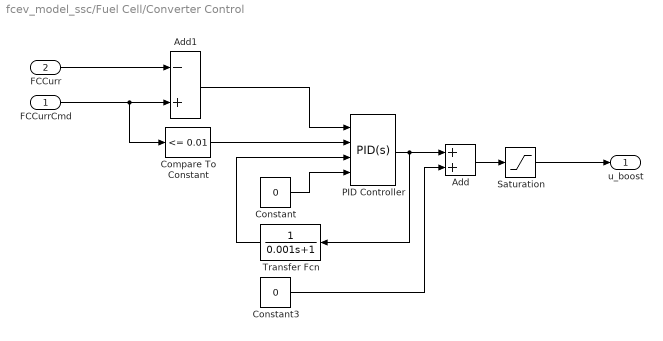
== system fcev_model_ssc/Fuel Cell/Converter Control ==
  FCCurrCmd : Inport
  FCCurr : Inport  Port=2
  Add : Sum
  Add1 : Sum  Inputs=-+
  Compare To Constant : simulink/Logic and Bit Operations/Compare To Constant  relop=<=  const=0.01  OutDataTypeStr=boolean  ZeroCross=off
  Constant : Constant  Value=0
  Constant3 : Constant  Value=0
  PID Controller : slpidlib/PID Controller  Controller=PID  Form=Parallel  TimeDomain=Continuous-time  UseExternalTs=off  SampleTime=-1  IntegratorMethod=Forward Euler  FilterMethod=Forward Euler  ControllerParametersSource=internal  P=0.006  I=0.01  UseKiTs=off  D=0  N=100  UseFilter=on  TunerSelectOption=Transfer Function Based (PID Tuner App)  InitialConditionSource=external  InitialConditionForIntegrator=0  InitialConditionForFilter=0  DifferentiatorICPrevScaledInput=0  ExternalReset=falling  TrackingMode=off  Kt=1  LimitOutput=on  SatLimitsSource=internal  UpperSaturationLimit=1  LowerSaturationLimit=-1  LinearizeAsGain=on  AntiWindupMode=none  Kb=1  LimitIntegrator=off  UpperIntegratorSaturationLimit=inf  LowerIntegratorSaturationLimit=-inf  POutMin=[]  POutMax=[]  IOutMin=[]  IOutMax=[]  DOutMin=[]  DOutMax=[]  NOutMin=[]  NOutMax=[]  SumOutMin=[]  SumOutMax=[]  SaturationOutMin=[]  SaturationOutMax=[]  PParamMin=[]  PParamMax=[]  IParamMin=[]  IParamMax=[]  DParamMin=[]  DParamMax=[]  NParamMin=[]  NParamMax=[]  KbParamMin=[]  KbParamMax=[]  KtParamMin=[]  KtParamMax=[]  KbOutMin=[]  KbOutMax=[]  KtOutMin=[]  KtOutMax=[]  IntegratorOutMin=[]  IntegratorOutMax=[]  FilterOutMin=[]  FilterOutMax=[]  SumI1OutMin=[]  SumI1OutMax=[]  SumI2OutMin=[]  SumI2OutMax=[]  SumI3OutMin=[]  SumI3OutMax=[]  SumI4OutMin=[]  SumI4OutMax=[]  SumDOutMin=[]  SumDOutMax=[]  DifferentiatorOutMin=[]  DifferentiatorOutMax=[]  FilterDiffOutCoefMin=[]  FilterDiffOutCoefMax=[]  ReciprocalOutMin=[]  ReciprocalOutMax=[]  SumDenOutMin=[]  SumDenOutMax=[]  SumNumOutMin=[]  SumNumOutMax=[]  DivideOutMin=[]  DivideOutMax=[]  UdiffTsProdOutMin=[]  UdiffTsProdOutMax=[]  NTsProdOutMin=[]  NTsProdOutMax=[]  UintegralTsProdOutMin=[]  UintegralTsProdOutMax=[]  UngainTsProdOutMin=[]  UngainTsProdOutMax=[]  ClampingZeroOutDataTypeStr=Inherit: Inherit via back propagation  ClampingZeroOutMin=[]  ClampingZeroOutMax=[]  FilterDenConstantOutDataTypeStr=Inherit: Inherit via back propagation  FilterDenConstantOutMin=[]  FilterDenConstantOutMax=[]  PCopyOutDataTypeStr=Inherit: Inherit via back propagation  PCopyOutMin=[]  PCopyOutMax=[]  NCopyOutDataTypeStr=Inherit: Inherit via back propagation  NCopyOutMin=[]  NCopyOutMax=[]  IntegratorContinuousStateAttributes=''  IntegratorStateMustResolveToSignalObject=off  IntegratorRTWStateStorageClass=Auto  FilterContinuousStateAttributes=''  FilterStateMustResolveToSignalObject=off  FilterRTWStateStorageClass=Auto  ParallelPVariant=InternalParameters  IdealPVariant=Disabled  IVariant=InternalParameters  DVariant=InternalParameters  IntegratorVariant=Continuous  SatVariant=Enabled  AWVariant=Passthrough  PCopyVariant=Disabled  TRVariant=Disabled  FdbkBlocksVariant=Forward  IdealPFdbkVariant=Disabled  SatFdbkVariant=Disabled  DerivativeFilterVariant=ContFilter  NVariant=InternalParameters  NCopyVariant=Disabled  FilterICVariant=ExternalICs  IntegratorICVariant=ExternalICs  ExternalResetVariant=ExternalReset  TRSumVariant=Passthrough  SumFdbkVariant=Disabled  SumVariant=Sum_PID  TsampFilterVariant=InternalTs  TsampNgainVariant=Passthrough  TsampIntegralVariant=Disabled_SignalSpec  ExternalSaturationOutDataTypeStr=Inherit: Same as second input
  Saturation : Saturate  UpperLimit=1  LowerLimit=0  ZeroCross=off
  Transfer Fcn : TransferFcn  Denominator=[0.001 1]
  u_boost : Outport
  wires:
  Constant3/1 -> Add/2
  PID Controller/1 -> Add/1, Transfer Fcn/1
  FCCurr/1 -> Add1/1
  Add/1 -> Saturation/1
  FCCurrCmd/1 -> Compare To Constant/1, Add1/2
  Add1/1 -> PID Controller/1
  Transfer Fcn/1 -> PID Controller/3
  Constant/1 -> PID Controller/4
  Compare To Constant/1 -> PID Controller/2
  Saturation/1 -> u_boost/1

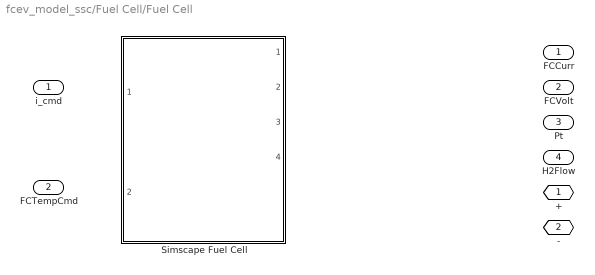
== system fcev_model_ssc/Fuel Cell/Fuel Cell ==
  i_cmd : Inport
  FCTempCmd : Inport  Port=2
  Simscape Fuel Cell : Subsystem  VariantControl=SimscapeFuelCell  ReferencedSubsystem=SSCFuelCell
  + : PMIOPort  Side=Right
  - : PMIOPort  Port=2  Side=Right
  FCCurr : Outport
  FCVolt : Outport  Port=2
  Pt : Outport  Port=3
  H2Flow : Outport  Port=4

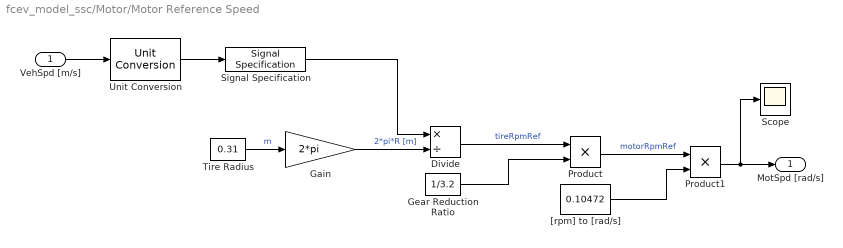
== system fcev_model_ssc/Motor/Motor Reference Speed ==
  VehSpd [m/s] : Inport
  Divide : Product  Inputs=*/
  Gain : Gain  Gain=2*pi
  Gear Reduction Ratio : Constant  Value=1/3.2
  Product : Product
  Product1 : Product
  Scope : Scope
  Signal Specification : SignalSpecification  Unit=m/min
  Tire Radius : Constant  Value=0.31
  Unit Conversion : UnitConversion
  "[rpm] to [rad/s]" : Constant  Value=0.10472
  MotSpd [rad/s] : Outport
  wires:
  VehSpd [m/s]/1 -> Unit Conversion/1
  Divide/1 -> Product/1  "tireRpmRef"
  Gain/1 -> Divide/2  "2*pi*R [m]"
  Gear Reduction Ratio/1 -> Product/2
  Tire Radius/1 -> Gain/1  "m"
  Product1/1 -> MotSpd [rad/s]/1, Scope/1
  "[rpm] to [rad/s]"/1 -> Product1/2
  Product/1 -> Product1/1  "motorRpmRef"
  Signal Specification/1 -> Divide/1
  Unit Conversion/1 -> Signal Specification/1

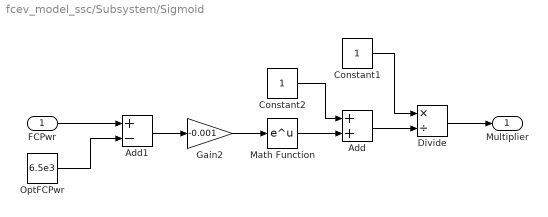
== system fcev_model_ssc/Subsystem/Sigmoid ==
  FCPwr : Inport
  Add : Sum
  Add1 : Sum  Inputs=+-
  Constant1 : Constant
  Constant2 : Constant
  Divide : Product  Inputs=*/
  Gain2 : Gain  Gain=-0.001
  Math Function : Math
  OptFCPwr : Constant  Value=6.5e3
  Multiplier : Outport
  wires:
  Add1/1 -> Gain2/1
  Divide/1 -> Multiplier/1
  Math Function/1 -> Add/2
  Add/1 -> Divide/2
  OptFCPwr/1 -> Add1/2
  Constant2/1 -> Add/1
  FCPwr/1 -> Add1/1
  Gain2/1 -> Math Function/1
  Constant1/1 -> Divide/1
